simulink model "s_2DOF_SOPDTUZ"  (R2018b)
settings: Solver=ode45  StartTime=0.0  StopTime=simT  MaxStep=Tsm  RelTol=rtol  AbsTol=atol
values from neighbouring files (symbols this model uses):
  D1 = [T^2 2*T 1]    [Figure_08.m]    (also in PD1nR_2DOF_Qn.m; PD3nR_2DOF_Qn.m; PD5nR_2DOF_Qn.m; PD7nR_2DOF_Qn.m)
  di0 = 0    [Figure_03a_above.m]    (also in Figure_03b_middle.m; Figure_03c_below.m; Figure_04.m; Figure_05.m)
  di1 = 1    [Figure_03a_above.m]    (also in Figure_03b_middle.m; Figure_03c_below.m; Figure_04.m; Figure_05.m)
  do = 0    [Figure_03a_above.m]    (also in Figure_03b_middle.m; Figure_03c_below.m; Figure_04.m; Figure_05.m)
  do0 = 0    [Figure_03a_above.m]    (also in Figure_03b_middle.m; Figure_03c_below.m; Figure_04.m; Figure_05.m)
  Dp = conv([Ti 1],[TD1 1])    [PD1nR_2DOF_Qn.m]    (also in PD3nR_2DOF_Qn.m = conv([Ti 1],[TD3  TD2 TD1 1]); PD5nR_2DOF_Qn.m = conv([Ti 1],[TD5 TD3  TD2 TD1 1]); PD7nR_2DOF_Qn.m = conv([Ti 1],[TD7 TD6 TD5 TD4 TD3 TD2 TD1 1]))
  dy = .1    (= 0.1)    [Figure_03a_above.m]    (also in Figure_03b_middle.m; Figure_03c_below.m; Figure_04.m = 0.05; Figure_05.m = 0.05)
  Kdy = 0    [Figure_03a_above.m]    (also in Figure_03b_middle.m; Figure_03c_below.m; Figure_04.m; Figure_05.m)
  N1 = K*[-T0 1]    [Figure_08.m]    (also in PD1nR_2DOF_Qn.m; PD3nR_2DOF_Qn.m; PD5nR_2DOF_Qn.m; PD7nR_2DOF_Qn.m)
  Nc = [Kd1 Kc]    [PD1nR_2DOF_Qn.m]    (also in PD1nR_NcPn.m; PD3nR_2DOF_Qn.m = [Kd3 Kd2 Kd1 Kc]; PD3nR_NcPn.m = [Kd3 Kd2 Kd1 Kc]; PD5nR_2DOF_Qn.m = [Kd5 Kd4 Kd3 Kd2 Kd1 Kc])
  ti = Ts    (= 0.001)    [Figure_03a_above.m]    (also in Figure_03b_middle.m; Figure_03c_below.m; Figure_04.m; Figure_05.m)
  Ti = taui*Td    [PD1nR_2DOF_Qn.m]    (also in PD1nR_NcPn.m; PD3nR_2DOF_Qn.m; PD3nR_NcPn.m; PD5nR_2DOF_Qn.m)
  to = Ts    (= 0.001)    [Figure_03a_above.m]    (also in Figure_03b_middle.m; Figure_03c_below.m; Figure_04.m; Figure_05.m)
  Ts = 0.001    [Figure_03a_above.m]    (also in Figure_03b_middle.m; Figure_03c_below.m; Figure_04.m; Figure_05.m)
  tw = Ts    (= 0.001)    [Figure_03a_above.m]    (also in Figure_03b_middle.m; Figure_03c_below.m; Figure_04.m; Figure_05.m)
  Umax = 10    [Figure_03a_above.m]    (also in Figure_03b_middle.m; Figure_03c_below.m; Figure_04.m; Figure_05.m)
  Umin = -10    [Figure_03a_above.m]    (also in Figure_03b_middle.m; Figure_03c_below.m; Figure_04.m; Figure_05.m)
  w0 = 0    [Figure_03a_above.m]    (also in Figure_03b_middle.m; Figure_03c_below.m; Figure_04.m; Figure_05.m)
  w1 = 0    [Figure_03a_above.m]    (also in Figure_03b_middle.m; Figure_03c_below.m; Figure_04.m; Figure_05.m)
undefined symbols (not defined in the file or in its folder): Np, Pn
settings Model: ExtModeTrigMode=oneshot  ExtModeArmWhenConnect=off  Creator=mhuba  LastModifiedBy=mhuba
settings SolverCC: AutoScaleAbsTol=off
settings DataIOCC: SaveFormat=Array  SignalLoggingSaveFormat=ModelDataLogs  SignalLoggingName=sigsOut
settings OptimizationCC: BooleanDataType=off  ExpressionDepthLimit=2147483647  LifeSpan=inf
settings DebuggingCC: SaveWithParameterizedLinksMsg=none  UnderspecifiedInitializationDetection=Classic  MergeDetectMultiDrivingBlocksExec=none  SignalResolutionControl=TryResolveAllWithWarning  MultiTaskDSMMsg=warning  MultiTaskCondExecSysMsg=none  FcnCallInpInsideContextMsg=warning  StateNameClashWarn=warning  SFUnexpectedBacktrackingDiag=warning  SFNoUnconditionalDefaultTransitionDiag=warning  SFExecutionAtInitializationDiag=none
settings HardwareCC: ProdBitPerPointer=32  ProdBitPerSizeT=32  ProdBitPerPtrDiffT=32  ProdLargestAtomicFloat=None  ProdIntDivRoundTo=Undefined  ProdEndianess=Unspecified  ProdWordSize=32  ProdHWDeviceType=32-bit Generic  TargetUnknown=on
settings ModelReferenceCC: PropagateSignalLabelsOutOfModel=off
settings SFSimCC: SimUseLocalCustomCode=off
settings RTWCC: TemplateMakefile=grt_vc.tmf  RTWUseLocalCustomCode=off
settings CodeAppCC: StateflowObjectComments=on
settings GRTTargetCC: TargetLangStandard=C89/C90 (ANSI)  CombineOutputUpdateFcns=off  GRTInterface=on
settings ConfigComp: CovMetricSettings=dw  CovSaveCumulativeToWorkspaceVar=on  CovSaveSingleToWorkspaceVar=on  CovExternalEMLEnable=off

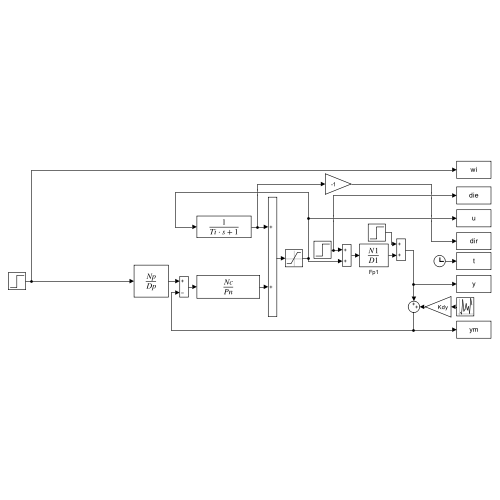
[thumbnail: Simulink's stored preview of the top-level diagram]
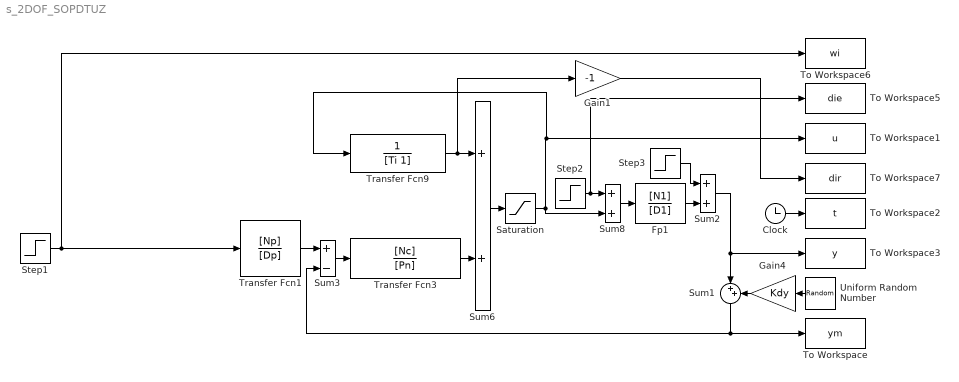
== system s_2DOF_SOPDTUZ ==
  Clock : Clock
  Fp1 : TransferFcn  Numerator=[N1]  Denominator=[D1]
  Gain1 : Gain  Gain=-1  SaturateOnIntegerOverflow=on  OutDataTypeStr=Inherit: Same as input  ParamDataTypeStr=Inherit: Same as input
  Gain4 : Gain  Gain=Kdy  SaturateOnIntegerOverflow=on  OutDataTypeStr=Inherit: Same as input  ParamDataTypeStr=Inherit: Same as input
  Saturation : Saturate  UpperLimit=Umax  LowerLimit=Umin
  Step1 : Step  Time=tw  Before=w0  After=w1  SampleTime=Ts
  Step2 : Step  Time=ti  Before=di0  After=di1  SampleTime=Ts
  Step3 : Step  Time=to  Before=do0  After=do  SampleTime=Ts
  Sum1 : Sum  Inputs=|++  InputSameDT=on  SaturateOnIntegerOverflow=on  OutDataTypeStr=Inherit: Same as first input
  Sum2 : Sum  InputSameDT=on  SaturateOnIntegerOverflow=on  OutDataTypeStr=Inherit: Same as first input
  Sum3 : Sum  Inputs=+-  InputSameDT=on  SaturateOnIntegerOverflow=on  OutDataTypeStr=Inherit: Same as first input
  Sum6 : Sum  InputSameDT=on  SaturateOnIntegerOverflow=on  OutDataTypeStr=Inherit: Same as first input
  Sum8 : Sum  InputSameDT=on  SaturateOnIntegerOverflow=on  OutDataTypeStr=Inherit: Same as first input
  To Workspace : ToWorkspace  VariableName=ym  SampleTime=Ts
  To Workspace1 : ToWorkspace  VariableName=u  SampleTime=Ts
  To Workspace2 : ToWorkspace  VariableName=t  SampleTime=Ts
  To Workspace3 : ToWorkspace  VariableName=y  SampleTime=Ts
  To Workspace5 : ToWorkspace  VariableName=die  SampleTime=Ts
  To Workspace6 : ToWorkspace  VariableName=wi  SampleTime=Ts
  To Workspace7 : ToWorkspace  VariableName=dir  SampleTime=Ts
  Transfer Fcn1 : TransferFcn  Numerator=[Np]  Denominator=[Dp]
  Transfer Fcn3 : TransferFcn  Numerator=[Nc]  Denominator=[Pn]
  Transfer Fcn9 : TransferFcn  Numerator=[1 ]  Denominator=[Ti 1]
  Uniform Random Number : UniformRandomNumber  Minimum=-dy  Maximum=dy  SampleTime=Ts
  wires:
  Step1/1 -> To Workspace6/1, Transfer Fcn1/1
  Sum8/1 -> Fp1/1
  Step2/1 -> Sum8/1, To Workspace5/1
  Clock/1 -> To Workspace2/1
  Sum2/1 -> Sum1/1, To Workspace3/1
  Uniform Random Number/1 -> Gain4/1
  Gain4/1 -> Sum1/2
  Step3/1 -> Sum2/1
  Fp1/1 -> Sum2/2
  Transfer Fcn1/1 -> Sum3/1
  Sum1/1 -> To Workspace/1, Sum3/2
  Transfer Fcn3/1 -> Sum6/2
  Transfer Fcn9/1 -> Gain1/1, Sum6/1
  Sum6/1 -> Saturation/1
  Saturation/1 -> Sum8/2, Transfer Fcn9/1, To Workspace1/1
  Sum3/1 -> Transfer Fcn3/1
  Gain1/1 -> To Workspace7/1
